simulink model "ev"  (R2021a)
settings: Solver=ode4  StartTime=0  StopTime=1082  FixedStep=sim_dt  RelTol=1e-3
model workspace (MAT data in the model file):
  T_eff_bp = [-270; -210; -150; -90; -30; 30; 90; 150; 210; 270]
  T_eff_bp_2 = [-270; -210; -150; -90; -30; 30; 90; 150; 210; 270]
  losses_table = [108927.107777 7820.2782368 7820.17609997 7820.2782368 7820.2782368 7820.2782368 7820.2782368 7820.26172359 7820.2782368 9345.38006027 108927.107777 7820.2782368 ... (100 elements, 10x10)]
  losses_table_2 = [108927.107777 7820.2782368 7820.17609997 7820.2782368 7820.2782368 7820.2782368 7820.2782368 7820.26172359 7820.2782368 9345.38006027 108927.107777 7820.2782368 ... (100 elements, 10x10)]
  w_eff_bp = [0; 888.888888889; 1777.77777778; 2666.66666667; 3555.55555556; 4444.44444444; 5333.33333333; 6222.22222222; 7111.11111111; 8000]
  w_eff_bp_2 = [0; 888.888888889; 1777.77777778; 2666.66666667; 3555.55555556; 4444.44444444; 5333.33333333; 6222.22222222; 7111.11111111; 8000]
undefined symbols (not defined in the file): Af, alpha, Bt, C, C_fa, C_free, C_sa_bat, C_sa_uc, Cd, Cmax, Continuous, Crr, DoD, effi, etaFD, etaG, FD, G, gear, Iucmax, m, M1m, M2m, Max, npar, npar_free, npara, nparf, nparfa, nparsa_bat, nparsa_UC, nser, nser_free, nserfa, nsersa_bat, nsersa_UC, Qbat, regenmax, Ri_BP, RL, ro, Rsc, Rsc_A, Rsc_F, Rsc_sa_bat, Rsc_sa_uc, rw, sim_dt, SOC_BP, SoCbatmax, SoCbatmin, SoCucmax, SoCucmin, speed, torque, VinBat, Voc_BP, Vuc, Vuc_fa, Vuc_free ... (+2)
libraries: autolibshared x41, simulink x26, autolibdcdc x13, autolibdatasheetbattery x7, autolibmappedmotor x6, fl_lib x3, nesl_utility x3, spsSupercapacitorLib x3, pid_lib x1
(part 18 of 18)

== matlab function ev/Drive cycle power demand/Controller. Actual motor torque/MATLAB Function ==
  data: trq_wh input; g1 output; w_wh input; P_veh input; Tau_def output; G parameter; effi parameter; speed parameter; torque parameter; etaG parameter; WG_def output; g0 input; gs output; Max parameter; Tmax output; Tmin output; Continuous parameter; g_prev input; n_mtr output; com output; test input; WG output; Vtest input; mode input; FD parameter; etaFD parameter; regenmax parameter
function [g1,Tau_def,WG_def,gs,Tmax,Tmin,n_mtr,com,WG] = fcn(trq_wh,w_wh,P_veh,G,effi, speed, torque,etaG,g0, Max,Continuous,g_prev,test,Vtest,mode,FD,etaFD,regenmax)



Wgb_out=w_wh.*FD;


WG=Wgb_out.*G; %Vel angular despues del Gear, ws intech velocidad angular de la flecha del motor el�ctrico ecuaci�n 8

WG(WG>max(Continuous(:,1))*pi/30)=max(Continuous(:,1))*pi/30;







    if P_veh>0
            Tgb_out=(1/etaFD)*trq_wh./(FD);
            Tau=(1/etaG)*Tgb_out./(G); %torque mecánico del motor electrico
                
           n_mtr=interp2(speed*(2*pi/60),-torque,effi,WG,Tau);
           if mode == 0 % for now the selection is only available with accel profile
            
            [com,gs]=min(WG); %for high performance mode 
           else
            [com,gs]=max(n_mtr); %for eco mode
           end
    else
            Tgb_out=(etaFD)*trq_wh./(FD);
            Tau=(etaG)*Tgb_out./(G);%torque mecnánico del generador electrico
                Tau(Tau<regenmax)=regenmax;
            n_mtr=interp2(speed*(2*pi/60),-torque,effi,WG,Tau);
            [com,gs]=max(n_mtr);
            
            
    %          gs=g_prev;
    %          com=n_mtr(:,gs);
    end

test1=all(test);

    if test1==1 % si los 30 anteriores son iguales

            if com==0
        
                gs=g_prev;
                WG_def=WG(gs);
                Tau_def=Tau(gs);
            else
                if Vtest==1 && g_prev>gs
                    
                    
                    gs=g_prev;
                    WG_def=WG(gs);
                    Tau_def=Tau(gs);
                else
                    gs=gs;
                    WG_def=WG(gs);
                    Tau_def=Tau(gs);
                end
            end
    Tmax=interp1(Continuous(:,1),Continuous(:,2),abs(WG_def)*(30/pi));
    Tmin=interp1(Continuous(:,1),-Continuous(:,2),abs(WG_def)*(30/pi));

    % Tcmax=interp1(Continuous(:,1),Continuous(:,2),WG_def*(30/pi));
    % Tcmin=interp1(Continuous(:,1),-Continuous(:,2),abs(WG_def)*(30/pi));

%         if     gs==1; 
%             g1=G(1);
%         elseif gs==2; 
%             g1=G(2);
% %         elseif gs==3; 
% %             g1=G(3);
% %         elseif gs==4; 
% %             g1=G(4);
% %         elseif gs==5; 
% %             g1=G(5);
% %         elseif gs==6; 
% %             g1=G(6);
% %         elseif gs==7; 
% %             g1=G(7);
% %         elseif gs==8; 
% %             g1=G(8); 
% %         else
%             g1=G(1);
%         end
        
%             g1=G(gs);
    else  %si el cambio de velocidad no ha sido constante los ultimos 30 dt
        gs=g_prev;
        WG_def=WG(gs);
        Tau_def=Tau(gs);  

    Tmax=interp1(Continuous(:,1),Continuous(:,2),abs(WG_def)*(30/pi));
    Tmin=interp1(Continuous(:,1),-Continuous(:,2),abs(WG_def)*(30/pi));

    % Tcmax=interp1(Continuous(:,1),Continuous(:,2),WG_def*(30/pi));
    % Tcmin=interp1(Continuous(:,1),-Continuous(:,2),abs(WG_def)*(30/pi));

%         if     gs==1; 
%             g1=G(1);
%         elseif gs==2; 
%             g1=G(2);
% %         elseif gs==3; 
% %             g1=G(3);
% %         elseif gs==4; 
% %             g1=G(4);
% %         elseif gs==5; 
% %             g1=G(5);
% %         elseif gs==6; 
% %             g1=G(6);
% %         elseif gs==7; 
% %             g1=G(7);
% %         elseif gs==8; 
% %             g1=G(8); 
%         else
%             g1=G(1);
%         end

            g1=G(gs);

    end
    
    
    
    
    

end

== matlab function ev/Tesis/HESS/Full active4/MATLAB Function3 ==
  data: Id output; Vo input; Vd input; eff input; Po input; Pd output; Io output
function [Id,Pd,Io]  = fcn(Vo,Vd,eff, Po)

if Po>0
    Pd=Po;
    Id=Pd/Vd;
    Io=Po/Vo;
elseif Po<0
    Pd=Po;
    Id=Pd/Vd;
    Io=Po/Vo;
else
    Pd=Po;
    Id=Pd/Vd;
    Io=Po/Vo;
end
   

end

== matlab function ev/Tesis/HESS/Full_active/MATLAB Function2 ==
  data: OCV input; I_batt output; Ri input; P input
function I_batt   = fcn(OCV,Ri,P)

%I_batt=(-OCV-sqrt((OCV^2)-(4*(-Ri)*(-P))))/(2*(-Ri));

I_batt=(-(OCV-(OCV^2-4*P*Ri)^(1/2))/(2*Ri));

% I_batt=roots([Ri -OCV P]);
% imIb=imag(I_batt);
% I_batt=min(imIb)
end

== matlab function ev/Tesis/HESS/Full active4/MATLAB Function5 ==
  data: Id output; Vo input; Vd input; eff input; Po input; Pd output; Io output
function [Id,Pd,Io]  = fcn(Vo,Vd,eff, Po)


    Pd=Po;
    Id=Pd/Vd;
    Io=Po/Vo;

   

end

== matlab function ev/Tesis/HESS/semi_active_UC/MATLAB Function ==
  data: Ireq output; Iout output; Preq input; V_bat input; V_uc input; Ibat output; Iuc output; SoCbat input; SoCuc input; err output; stop output; test input; flagpow output; mode output; convDCDC input; conDCDC input; Qbat parameter; nparsa_UC parameter; Iucmax parameter; npara parameter; SoCbatmin parameter; SoCucmin parameter; SoCbatmax parameter; SoCucmax parameter; Cmax parameter; Pdispm output; Pdispn output
function [Ireq,Iout,Ibat,Iuc,err,stop,flagpow,mode,Pdispm,Pdispn] = fcn(Preq,V_bat,V_uc,SoCbat,SoCuc,test,convDCDC,conDCDC,Qbat, nparsa_UC, Iucmax, npara, SoCbatmin, SoCucmin, SoCbatmax, SoCucmax,Cmax)

% if V_bat==V_uc
    V_tot=V_bat;
% else
%     V_tot=V_uc;
% end


Ireq=(Preq/V_tot);

Ibatdis=Qbat*nparsa_UC*Cmax;
Ibatcha=-Qbat*nparsa_UC*Cmax;

Pbatcha=Ibatcha*V_bat;%*convDCDC;
Pbatdis=Ibatdis*V_bat;%*convDCDC;

Iucdis=Iucmax*npara;
Iuccha=-Iucmax*npara;

Puccha=Iuccha*V_uc;%*conDCDC;
Pucdis=Iucdis*V_uc;%*conDCDC;

Pdispm=Pbatdis+Pucdis;
Pdispn=Pbatcha+Puccha;


   if Preq==0
       mode=0;
   elseif Preq>0
       if Preq<=(Pucdis+Pbatdis)
          if SoCbat<=SoCbatmin
              if SoCuc<=SoCucmin
                  mode=1;
              else
                  if Iucdis*convDCDC>=Ireq
                      mode=2;
                  else
                      mode=3;
                  end
              end
          else
              if SoCuc<=SoCucmin
                  if Ibatdis*convDCDC>=Ireq
                      mode=4;
                  else
                      mode=5;
                  end
              else
                  if test>0
                      if Iucdis*conDCDC>=Ireq
                          mode=6;
                      else
                          mode=7;
                      end
                  elseif test<0
                      if Ibatdis*convDCDC>=Ireq
                          mode=8;
                      else
                          mode=9;
                      end
                  else
                      mode=25;
                  end
              end
          end
       else
           if SoCbat<=SoCbatmin
               if SoCuc<=SoCucmin
                   mode=10;
               else
                   mode=11;
               end
           else
               if SoCuc<=SoCucmin
                   mode=12;
               else
                   mode=13;
               end
           end
       end
   elseif Preq<0
       if Preq>=(Pdispn)
           if SoCuc<=SoCucmax
               if SoCbat<=SoCbatmax
                   if Iuccha*conDCDC>=Ireq
                       mode=14;
                   else
                       mode=15;
                   end
               else
                   if Iuccha*conDCDC>Ireq
                       mode=16;
                   else
                       mode=17;
                   end
               end
           else
               if SoCbat<=SoCbatmax
                   if Ibatcha*convDCDC>Ireq
                       mode=18;
                   else
                       mode=19;
                   end
               else
                   mode=20;
               end
           end
       else
           if SoCuc<=SoCucmax
               if SoCbat<=SoCbatmax
                   mode=21;
               else
                   mode=22;
               end
           else
               if SoCbat<=SoCbatmax
                   mode=23;
               else
                   mode=24;
               end
           end
       end
   else
       mode=26;
   end
   
   switch mode
       case 0
           Iuc=0;
           Ibat=0;
           stop=0;
           err=0;
           flagpow=0;           
       case 1
           Iuc=0;
           Ibat=0;
           stop=1;
           err=0;
           flagpow=0;
       case 2
           Iuc=Ireq;
           Ibat=0;
           stop=0;
           err=0;
           flagpow=0;
       case 3
           Iuc=Iucdis*conDCDC;
           Ibat=0;
           stop=0;
           err=0;
           flagpow=1;
       case 4
           Iuc=Ireq-Ibatdis*convDCDC;
           Ibat=Ibatdis*convDCDC;
           stop=0;
           err=0;
           flagpow=0;
       case 5
           Iuc=0;
           Ibat=Ibatdis*convDCDC;
           stop=0;
           err=0;
           flagpow=1;
       case 6
           Iuc=Ireq;
           Ibat=0;
           stop=0;
           err=0;
           flagpow=0;
       case 7
           Iuc=Iucdis*conDCDC;
           Ibat=Ireq-Iucdis*conDCDC;
           stop=0;
           err=0;
           flagpow=0;
       case 8
           Iuc=Ireq-Ibatdis*convDCDC;
           Ibat=Ibatdis*convDCDC;
           stop=0;
           err=0;
           flagpow=0;
       case 9
           Iuc=0;
           Ibat=Ibatdis*convDCDC;
           stop=0;
           err=0;
           flagpow=1;
       case 10
           Iuc=0;
           Ibat=0;
           stop=1;
           err=0;
           flagpow=1;
       case 11
           Iuc=Iucdis*conDCDC;
           Ibat=0;
           stop=0;
           err=0;
           flagpow=1;
       case 12
           Iuc=0;
           Ibat=Ibatdis*convDCDC;
           stop=0;
           err=0;
           flagpow=1;
       case 13
           Iuc=Iucdis*conDCDC;
           Ibat=Ibatdis*convDCDC;
           stop=0;
           err=0;
           flagpow=1;
       case 14
           Iuc=Iuccha*conDCDC;;
           Ibat=Ireq-Iuccha*conDCDC;
           stop=0;
           err=0;
           flagpow=0;
       case 15 %mod
           Iuc=Ireq;
           Ibat=0;
           stop=0;
           err=0;
           flagpow=0;
       case 16
           Iuc=Iuccha*conDCDC;
           Ibat=0;
           stop=0;
           err=0;
           flagpow=1;
       case 17
           Iuc=Ireq;
           Ibat=0;
           stop=0;
           err=0;
           flagpow=0;
       case 18
           Iuc=0;
           Ibat=Ibatcha*convDCDC;
           stop=0;
           err=0;
           flagpow=0;
       case 19 %mod
           Iuc=0;
           Ibat=Ireq;
           stop=0;
           err=0;
           flagpow=0;
       case 20
           Iuc=0;
           Ibat=0;
           stop=0;
           err=0;
           flagpow=1;
       case 21
           Iuc=Iuccha*conDCDC;
           Ibat=Ibatcha*convDCDC;
           stop=0;
           err=0;
           flagpow=1;
       case 22
           Iuc=Iuccha*conDCDC;
           Ibat=0;
           stop=0;
           err=0;
           flagpow=1;
       case 23
           Iuc=0;
           Ibat=Ibatcha*convDCDC;
           stop=0;
           err=0;
           flagpow=1;
       case 24
           Iuc=0;
           Ibat=0;
           stop=0;
           err=0;
           flagpow=1;
       case 25 %case when count is 0
           Iuc=0;
           Ibat=0;
           stop=0;
           err=1;
           flagpow=0;
       case 26 %¿? it should not exist
           Iuc=0;
           Ibat=0;
           stop=0;
           err=2;
           flagpow=0;
       otherwise
           Iuc=0;
           Ibat=0;
           stop=0;
           err=3;
           flagpow=0;
           mode=27;
   end
   Iuc=Iuc*1;
   Ibat=Ibat*1;
Iout=Iuc+Ibat;

end

== matlab function ev/Tesis/HESS/semi_active_bat/MATLAB Function1 ==
  data: SoCuc input; acurr output; bcurr output; mo1 output; mo2 output; aprev input; bprev input; count output; cprev input; a output; b output; test output; counta output; countb output; cpreva input; cprevb input; countc output
function [acurr,bcurr,mo1,mo2,count,a,b,test,counta,countb,countc] = fcn(SoCuc,aprev,bprev,cprev,cpreva,cprevb)

if SoCuc>=0.2
    acurr=0;
    mo1=1;
else
    acurr=1;
    mo1=2;
end
if SoCuc>=0.9
    bcurr=1;
    mo2=1;
else
    bcurr=0;
    mo2=2;
end

a=acurr-aprev;
b=bcurr-bprev;




if a==1 || b==1
%     count=cprev+a+b;
    counta=cpreva+a;
    countb=cprevb+b;
else
%     count=cprev;
    counta=cpreva;
    countb=cprevb;
end
countc=countb-counta;

if countc>0
    count=2;
else 
    count=1;
end

test=(-1)^(count);

end

== matlab function ev/Tesis/HESS/semi_active_UC/MATLAB Function2 ==
  data: OCV input; I_batt output; Ri input; P input
function I_batt   = fcn(OCV,Ri,P)

%I_batt=(-OCV-sqrt((OCV^2)-(4*(-Ri)*(-P))))/(2*(-Ri));

I_batt=(-(OCV-(OCV^2-4*P*Ri)^(1/2))/(2*Ri));

% I_batt=roots([Ri -OCV P]);
% imIb=imag(I_batt);
% I_batt=min(imIb)
end

== matlab function ev/Tesis/HESS/semi_active_UC/MATLAB Function3 ==
  data: Id output; Vo input; Vd input; eff input; Po input; Pd output; Io output
function [Id,Pd,Io]  = fcn(Vo,Vd,eff, Po)

if Po>0
    Pd=Po;
    Id=Pd/Vd;
    Io=Po/Vo;
elseif Po<0
    Pd=Po;
    Id=Pd/Vd;
    Io=Po/Vo;
else
    Pd=Po;
    Id=Pd/Vd;
    Io=Po/Vo;
end
   

end

== matlab function ev/Tesis/HESS/semi_active_bat/MATLAB Function ==
  data: Ireq output; Iout output; Preq input; V_bat input; V_uc input; Ibat output; Iuc output; SoCbat input; SoCuc input; err output; stop output; test input; flagpow output; mode output; convDCDC input; conDCDC input; Qbat parameter; nparsa_bat parameter; Iucmax parameter; nparf parameter; SoCucmin parameter; SoCbatmin parameter; SoCbatmax parameter; SoCucmax parameter; Cmax parameter
function [Ireq,Iout,Ibat,Iuc,err,stop,flagpow,mode] = fcn(Preq,V_bat,V_uc,SoCbat,SoCuc,test,convDCDC,conDCDC,Qbat, nparsa_bat, Iucmax, nparf, SoCucmin, SoCbatmin, SoCbatmax, SoCucmax,Cmax)

% if V_bat==V_uc
%     V_tot=V_bat;
% else
    V_tot=V_uc;
% end


Ireq=(Preq/V_tot);

Ibatdis=Qbat*nparsa_bat*Cmax;
Ibatcha=-Qbat*nparsa_bat*Cmax;

Pbatcha=Ibatcha*V_bat;%*convDCDC;
Pbatdis=Ibatdis*V_bat;%*convDCDC;

Iucdis=Iucmax*nparf;
Iuccha=-Iucmax*nparf;

Puccha=Iuccha*V_uc;%*conDCDC;
Pucdis=Iucdis*V_uc;%*conDCDC;




   if Preq==0
       mode=0;
   elseif Preq>0
       if Preq<=(Pucdis+Pbatdis)
          if SoCbat<=SoCbatmin
              if SoCuc<=SoCucmin
                  mode=1;
              else
                  if Iucdis*convDCDC>=Ireq
                      mode=2;
                  else
                      mode=3;
                  end
              end
          else
              if SoCuc<=SoCucmin
                  if Ibatdis*convDCDC>=Ireq
                      mode=4;
                  else
                      mode=5;
                  end
              else
                  if test>0
                      if Iucdis*conDCDC>=Ireq
                          mode=6;
                      else
                          mode=7;
                      end
                  elseif test<0
                      if Ibatdis*convDCDC>=Ireq
                          mode=8;
                      else
                          mode=9;
                      end
                  else
                      mode=25;
                  end
              end
          end
       else
           if SoCbat<=SoCbatmin
               if SoCuc<=SoCucmin
                   mode=10;
               else
                   mode=11;
               end
           else
               if SoCuc<=SoCucmin
                   mode=12;
               else
                   mode=13;
               end
           end
       end
   elseif Preq<0
       if Preq>=(Puccha+Pbatcha)
           if SoCuc<=SoCucmax
               if SoCbat<=SoCbatmax
                   if Iuccha*conDCDC>Ireq
                       mode=14;
                   else
                       mode=15;
                   end
               else
                   if Iuccha*conDCDC>Ireq
                       mode=16;
                   else
                       mode=17;
                   end
               end
           else
               if SoCbat<=SoCbatmax
                   if Ibatcha*convDCDC>Ireq
                       mode=18;
                   else
                       mode=19;
                   end
               else
                   mode=20;
               end
           end
       else
           if SoCuc<=SoCucmax
               if SoCbat<=SoCbatmax
                   mode=21;
               else
                   mode=22;
               end
           else
               if SoCbat<=SoCbatmax
                   mode=23;
               else
                   mode=24;
               end
           end
       end
   else
       mode=26;
   end
   
   switch mode
       case 0
           Iuc=0;
           Ibat=0;
           stop=0;
           err=0;
           flagpow=0;           
       case 1
           Iuc=0;
           Ibat=0;
           stop=1;
           err=0;
           flagpow=0;
       case 2
           Iuc=Ireq;
           Ibat=0;
           stop=0;
           err=0;
           flagpow=0;
       case 3
           Iuc=Iucdis*conDCDC;
           Ibat=0;
           stop=0;
           err=0;
           flagpow=1;
       case 4
           Iuc=Ireq-Ibatdis*convDCDC;
           Ibat=Ibatdis*convDCDC;
           stop=0;
           err=0;
           flagpow=0;
       case 5
           Iuc=0;
           Ibat=Ibatdis*convDCDC;
           stop=0;
           err=0;
           flagpow=1;
       case 6
           Iuc=Ireq;
           Ibat=0;
           stop=0;
           err=0;
           flagpow=0;
       case 7
           Iuc=Iucdis*conDCDC;
           Ibat=Ireq-Iucdis*conDCDC;
           stop=0;
           err=0;
           flagpow=0;
       case 8
           Iuc=Ireq-Ibatdis*convDCDC;
           Ibat=Ibatdis*convDCDC;
           stop=0;
           err=0;
           flagpow=0;
       case 9
           Iuc=0;
           Ibat=Ibatdis*convDCDC;
           stop=0;
           err=0;
           flagpow=1;
       case 10
           Iuc=0;
           Ibat=0;
           stop=1;
           err=0;
           flagpow=1;
       case 11
           Iuc=Iucdis*conDCDC;
           Ibat=0;
           stop=0;
           err=0;
           flagpow=1;
       case 12
           Iuc=0;
           Ibat=Ibatdis*convDCDC;
           stop=0;
           err=0;
           flagpow=1;
       case 13
           Iuc=Iucdis*conDCDC;
           Ibat=Ibatdis*convDCDC;
           stop=0;
           err=0;
           flagpow=1;
       case 14
           Iuc=Iuccha*conDCDC;;
           Ibat=Ireq-Iuccha*conDCDC;
           stop=0;
           err=0;
           flagpow=0;
       case 15 %mod
           Iuc=Ireq;
           Ibat=0;
           stop=0;
           err=0;
           flagpow=0;
       case 16
           Iuc=Iuccha*conDCDC;
           Ibat=0;
           stop=0;
           err=0;
           flagpow=1;
       case 17
           Iuc=Ireq;
           Ibat=0;
           stop=0;
           err=0;
           flagpow=0;
       case 18
           Iuc=0;
           Ibat=Ibatcha*convDCDC;
           stop=0;
           err=0;
           flagpow=0;
       case 19 %mod
           Iuc=0;
           Ibat=Ireq;
           stop=0;
           err=0;
           flagpow=0;
       case 20
           Iuc=0;
           Ibat=0;
           stop=0;
           err=0;
           flagpow=1;
       case 21
           Iuc=Iuccha*conDCDC;
           Ibat=Ibatcha*convDCDC;
           stop=0;
           err=0;
           flagpow=1;
       case 22
           Iuc=Iuccha*conDCDC;
           Ibat=0;
           stop=0;
           err=0;
           flagpow=1;
       case 23
           Iuc=0;
           Ibat=Ibatcha*convDCDC;
           stop=0;
           err=0;
           flagpow=1;
       case 24
           Iuc=0;
           Ibat=0;
           stop=0;
           err=0;
           flagpow=1;
       case 25 %case when count is 0
           Iuc=0;
           Ibat=0;
           stop=0;
           err=1;
           flagpow=0;
       case 26 %¿? it should not exist
           Iuc=0;
           Ibat=0;
           stop=0;
           err=2;
           flagpow=0;
       otherwise
           Iuc=0;
           Ibat=0;
           stop=0;
           err=3;
           flagpow=0;
           mode=27;
   end
   Iuc=Iuc*1;
   Ibat=Ibat*1;
Iout=Iuc+Ibat;

end

== matlab function ev/Tesis/HESS/Free/MATLAB Function ==
  data: Ireq output; Iout output; Preq input; V_bat input; V_uc input; Ibat output; I_uc output; SoCbat input; SoCuc input; err output; stop output; test input; flagpow output; mode output; convDCDC input; conDCDC input; Qbat parameter; npar_free parameter; Iucmax parameter; nparf parameter; SoCbatmin parameter; SoCucmin parameter; SoCbatmax parameter; SoCucmax parameter
function [Ireq,Iout,Ibat,I_uc,err,stop,flagpow,mode] = fcn(Preq,V_bat,V_uc,SoCbat,SoCuc,test,convDCDC,conDCDC,Qbat, npar_free, Iucmax, nparf, SoCbatmin, SoCucmin, SoCbatmax, SoCucmax)


    V_tot=V_bat;



Ireq=(Preq/V_tot);

Ibatdis=Qbat*npar_free;
Ibatcha=-Qbat*npar_free;

Pbatcha=Ibatcha*V_tot;%*convDCDC;
Pbatdis=Ibatdis*V_tot;%*convDCDC;

Iucdis=Iucmax*nparf;
Iuccha=-Iucmax*nparf;

Puccha=Iuccha*V_tot;%*conDCDC;
Pucdis=Iucdis*V_tot;%*conDCDC;



   
if V_bat==V_uc
        I_uc=Ireq/2;
        Ibat=Ireq/2;
        stop=0;
        err=0;
        flagpow=0;
        mode=0;
elseif V_bat>V_uc
        if Preq>=0
            if Preq<Pbatdis
            I_uc=Ireq-Ibatdis;
            Ibat=Ibatdis;
            stop=0;
            err=0;
            flagpow=0;
            mode=1;
            else
            I_uc=0;
            Ibat=Ibatdis;
            stop=0;
            err=0;
            flagpow=1;
            mode=2;
            end
        else  %si la potencia requerida es menor a cero
            if Preq<Puccha
            I_uc=Iuccha;
            Ibat=Ireq-Iuccha;
            stop=0;
            err=0;
            flagpow=0;
            mode=3;
            else
            I_uc=Ireq;
            Ibat=0;
            stop=0;
            err=0;
            flagpow=1;
            mode=4;
            end
        end
elseif V_bat<V_uc
        if Preq>0
            if Preq<=Pucdis  %la potencia total la puede dar el UC, tambien puede cargar la bateria
            I_uc=Ireq;
            Ibat=0;
            stop=0;
            err=0;
            flagpow=0;
            mode=5;
            else
            I_uc=Iucdis;
            Ibat=Ireq-Iucdis;
            stop=0;
            err=0;
            flagpow=1;
            mode=6;
            end
        elseif Preq<0
            if Preq<Puccha
            I_uc=Iuccha;
            Ibat=Ireq-Iuccha;
            stop=0;
            err=0;
            flagpow=0;
            mode=7;
            else
            I_uc=Ireq;
            Ibat=0;
            stop=0;
            err=0;
            flagpow=1;
            mode=8;
            end
        else
            I_uc=0;
            Ibat=0;
            stop=0;
            err=0;
            flagpow=0;
            mode=9;
        end
else
        I_uc=0;
        Ibat=0;
        stop=0;
        err=1;
        flagpow=0;
        mode=10;
    
end

    I_uc=I_uc*1;
    Ibat=Ibat*1;
    Iout=I_uc+Ibat;


end

== matlab function ev/Tesis/HESS/semi_active_bat/MATLAB Function2 ==
  data: OCV input; I_batt output; Ri input; P input
function I_batt   = fcn(OCV,Ri,P)

%I_batt=(-OCV-sqrt((OCV^2)-(4*(-Ri)*(-P))))/(2*(-Ri));

I_batt=(-(OCV-(OCV^2-4*P*Ri)^(1/2))/(2*Ri));

% I_batt=roots([Ri -OCV P]);
% imIb=imag(I_batt);
% I_batt=min(imIb)
end

== matlab function ev/Tesis/HESS/semi_active_UC/MATLAB Function4 ==
  data: SoCuc input; acurr output; bcurr output; mo1 output; mo2 output; aprev input; bprev input; count output; cprev input; a output; b output; test output; counta output; countb output; cpreva input; cprevb input; countc output
function [acurr,bcurr,mo1,mo2,count,a,b,test,counta,countb,countc] = fcn(SoCuc,aprev,bprev,cprev,cpreva,cprevb)

if SoCuc>=0.2
    acurr=0;
    mo1=1;
else
    acurr=1;
    mo1=2;
end
if SoCuc>=0.9
    bcurr=1;
    mo2=1;
else
    bcurr=0;
    mo2=2;
end

a=acurr-aprev;
b=bcurr-bprev;




if a==1 || b==1
%     count=cprev+a+b;
    counta=cpreva+a;
    countb=cprevb+b;
else
%     count=cprev;
    counta=cpreva;
    countb=cprevb;
end
countc=countb-counta;

if countc>0
    count=2;
else 
    count=1;
end

test=(-1)^(count);

end

== matlab function ev/Tesis/HESS/semi_active_bat/MATLAB Function5 ==
  data: Id output; Vo input; Vd input; eff input; Po input; Pd output; Io output
function [Id,Pd,Io]  = fcn(Vo,Vd,eff, Po)

if Po>0
    Pd=Po;
    Id=Pd/Vd;
    Io=Po/Vo;
elseif Po<0
    Pd=Po;
    Id=Pd/Vd;
    Io=Po/Vo;
else
    Pd=Po;
    Id=Pd/Vd;
    Io=Po/Vo;
end
   

end

== matlab function ev/Tesis/HESS/Free/MATLAB Function1 ==
  data: SoCuc input; acurr output; bcurr output; mo1 output; mo2 output; aprev input; bprev input; count output; cprev input; a output; b output; test output; counta output; countb output; cpreva input; cprevb input; countc output
function [acurr,bcurr,mo1,mo2,count,a,b,test,counta,countb,countc] = fcn(SoCuc,aprev,bprev,cprev,cpreva,cprevb)

if SoCuc>=0.2
    acurr=0;
    mo1=1;
else
    acurr=1;
    mo1=2;
end
if SoCuc>=0.9
    bcurr=1;
    mo2=1;
else
    bcurr=0;
    mo2=2;
end

a=acurr-aprev;
b=bcurr-bprev;




if a==1 || b==1
%     count=cprev+a+b;
    counta=cpreva+a;
    countb=cprevb+b;
else
%     count=cprev;
    counta=cpreva;
    countb=cprevb;
end
countc=countb-counta;

if countc>0
    count=2;
else 
    count=1;
end

test=(-1)^(count);

end

== matlab function ev/Tesis/HESS/Free/MATLAB Function2 ==
  data: OCV input; I_batt output; Ri input; P input
function I_batt   = fcn(OCV,Ri,P)

%I_batt=(-OCV-sqrt((OCV^2)-(4*(-Ri)*(-P))))/(2*(-Ri));

I_batt=(-(OCV-(OCV^2-4*P*Ri)^(1/2))/(2*Ri));

% I_batt=roots([Ri -OCV P]);
% imIb=imag(I_batt);
% I_batt=min(imIb)
end

== matlab function ev/Tesis/HESS/semi_active_bat/vehicle dynamics/MATLAB Function ==
  data: F_FA input; F_veh input; igu input; u output; velo input; z1 input; a output
function [u,a]  = fcn(F_FA,F_veh,igu,velo,z1)




if (F_FA-F_veh)<3 && (F_FA-F_veh)> (-3) 
    
    u=velo;
    a=1;
else
    a=0;
    u=z1;
end






end

== matlab function ev/Tesis/HESS/semi_active_UC/vehicle dynamics/MATLAB Function ==
  data: F_FA input; F_veh input; igu input; u output; velo input; z1 input; a output
function [u,a]  = fcn(F_FA,F_veh,igu,velo,z1)




if (F_FA-F_veh)<3 && (F_FA-F_veh)> (-3) 
    
    u=velo;
    a=1;
else
    a=0;
    u=z1;
end






end

== matlab function ev/Tesis/HESS/Full_active/vehicle dynamics/MATLAB Function ==
  data: F_FA input; F_veh input; igu input; u output; velo input; z1 input; a output
function [u,a]  = fcn(F_FA,F_veh,igu,velo,z1)




if (F_FA-F_veh)<3 && (F_FA-F_veh)> (-3) 
    
    u=velo;
    a=1;
else
    a=0;
    u=z1;
end






end

== matlab function ev/Tesis/HESS/Free/vehicle dynamics/MATLAB Function ==
  data: F_FA input; F_veh input; igu input; u output; velo input; z1 input; a output
function [u,a]  = fcn(F_FA,F_veh,igu,velo,z1)




if (F_FA-F_veh)<3 && (F_FA-F_veh)> (-3) 
    
    u=velo;
    a=1;
else
    a=0;
    u=z1;
end






end

== matlab function ev/Tesis/Battery model/MATLAB Function1 ==
  data: Ri input; Vb output; Ib input; Pmot input
function Vb = fcn(Ri,Ib,Pmot)

Vb=(((Ri*(Ib^2))+Pmot)/(Ib));


end

== matlab function ev/battery model limited/MATLAB Function ==
  data: OCV input; I_batt output; Ri input; P input
function I_batt   = fcn(OCV,Ri,P)

%I_batt=(-OCV-sqrt((OCV^2)-(4*(-Ri)*(-P))))/(2*(-Ri));

I_batt=(-(OCV-(OCV^2-4*P*Ri)^(1/2))/(2*Ri));

% I_batt=roots([Ri -OCV P]);
% imIb=imag(I_batt);
% I_batt=min(imIb)
end

== matlab function ev/battery model limited/MATLAB Function2 ==
  data: Ri input; Vb output; Ib input; Pmot input
function Vb = fcn(Ri,Ib,Pmot)

Vb=-(((Ri*(Ib^2))+Pmot)/(Ib));

Vb=Vb-Ri*Ib;

end

== matlab function ev/Tesis/HESS/Battery model/MATLAB Function1 ==
  data: Ri input; Vb output; Ib input; Pmot input
function Vb = fcn(Ri,Ib,Pmot)

Vb=(((Ri*(Ib^2))+Pmot)/(Ib));


end

== matlab function ev/Tesis/battery model limitedmod/MATLAB Function ==
  data: OCV input; I_batt output; Ri input; P input
function I_batt   = fcn(OCV,Ri,P)

%I_batt=(-OCV-sqrt((OCV^2)-(4*(-Ri)*(-P))))/(2*(-Ri));

I_batt=(-(OCV-(OCV^2-4*P*Ri)^(1/2))/(2*Ri));

% I_batt=roots([Ri -OCV P]);
% imIb=imag(I_batt);
% I_batt=min(imIb)
end

== matlab function ev/vehicle dynamics1/MATLAB Function ==
  data: F_FA input; F_veh input; igu input; u output; velo input; z1 input; a output
function [u,a]  = fcn(F_FA,F_veh,igu,velo,z1)




if (F_FA-F_veh)<3 && (F_FA-F_veh)> (-3) 
    
    u=velo;
    a=1;
else
    a=0;
    u=z1;
end






end

== matlab function ev/Tesis/Battery model/vehicle dynamics/MATLAB Function ==
  data: F_FA input; F_veh input; igu input; u output; velo input; z1 input; a output
function [u,a]  = fcn(F_FA,F_veh,igu,velo,z1)




if (F_FA-F_veh)<3 && (F_FA-F_veh)> (-3) 
    
    u=velo;
    a=1;
else
    a=0;
    u=z1;
end






end

== matlab function ev/Tesis/battery model limitedmod/MATLAB Function2 ==
  data: Ri input; Vb output; Ib input; Pmot input
function Vb = fcn(Ri,Ib,Pmot)

Vb=-(((Ri*(Ib^2))+Pmot)/(Ib));

Vb=Vb-Ri*Ib;

end

== matlab function ev/Tesis/HESS/battery model limited/MATLAB Function2 ==
  data: Ri input; Vb output; Ib input; Pmot input
function Vb = fcn(Ri,Ib,Pmot)

Vb=-(((Ri*(Ib^2))+Pmot)/(Ib));


end

== matlab function ev/Tesis/HESS/semi active Bat//Bat/MATLAB Function ==
  data: Ireq output; Iout output; Preq input; V_bat input; V_uc input; Ibat output; Iuc output; SoCbat input; SoCuc input; err output; stop output; test input; flagpow output; mode output; convDCDC input
function [Ireq,Iout,Ibat,Iuc,err,stop,flagpow,mode] = fcn(Preq,V_bat,V_uc,SoCbat,SoCuc,test,convDCDC)
conDCDC=1;
if V_bat==V_uc
    V_tot=V_bat;
else
    V_tot=V_uc;
end


Ireq=(Preq/V_tot);
Ibatdis=150;
Ibatcha=-150;
Pbatcha=Ibatcha*V_tot*convDCDC;
Pbatdis=Ibatdis*V_tot*convDCDC;
Iucdis=300;
Iuccha=-300;
Puccha=Iuccha*V_tot*conDCDC;
Pucdis=Iucdis*V_tot*conDCDC;


SoCbatmin=0.2;
SoCucmin=0.2;
SoCbatmax=0.85;
SoCucmax=0.95;




   if Preq==0
       mode=0;
   elseif Preq>0
       if Preq<=(Pucdis+Pbatdis)
          if SoCbat<=SoCbatmin
              if SoCuc<=SoCucmin
                  mode=1;
              else
                  if Iucdis>=Ireq
                      mode=2;
                  else
                      mode=3;
                  end
              end
          else
              if SoCuc<=SoCucmin
                  if Ibatdis*convDCDC>=Ireq
                      mode=4;
                  else
                      mode=5;
                  end
              else
                  if test>0
                      if Iucdis*conDCDC>=Ireq
                          mode=6;
                      else
                          mode=7;
                      end
                  elseif test<0
                      if Ibatdis*convDCDC>=Ireq
                          mode=8;
                      else
                          mode=9;
                      end
                  else
                      mode=25;
                  end
              end
          end
       else
           if SoCbat<=SoCbatmin
               if SoCuc<=SoCucmin
                   mode=10;
               else
                   mode=11;
               end
           else
               if SoCuc<=SoCucmin
                   mode=12;
               else
                   mode=13;
               end
           end
       end
   elseif Preq<0
       if Preq>=(Puccha+Pbatcha)
           if SoCuc<=SoCucmax
               if SoCbat<=SoCbatmax
                   if Iuccha*conDCDC>Ireq
                       mode=14;
                   else
                       mode=15;
                   end
               else
                   if Iuccha*conDCDC>Ireq
                       mode=16;
                   else
                       mode=17;
                   end
               end
           else
               if SoCbat<=SoCbatmax
                   if Ibatcha*convDCDC>Ireq
                       mode=18;
                   else
                       mode=19;
                   end
               else
                   mode=20;
               end
           end
       else
           if SoCuc<=SoCucmax
               if SoCbat<=SoCbatmax
                   mode=21;
               else
                   mode=22;
               end
           else
               if SoCbat<=SoCbatmax
                   mode=23;
               else
                   mode=24;
               end
           end
       end
   else
       mode=26;
   end
   
   switch mode
       case 0
           Iuc=0;
           Ibat=0;
           stop=0;
           err=0;
           flagpow=0;           
       case 1
           Iuc=0;
           Ibat=0;
           stop=1;
           err=0;
           flagpow=0;
       case 2
           Iuc=Ireq;
           Ibat=0;
           stop=0;
           err=0;
           flagpow=0;
       case 3
           Iuc=Iucdis*conDCDC;
           Ibat=0;
           stop=0;
           err=0;
           flagpow=1;
       case 4
           Iuc=Ireq-Ibatdis*convDCDC;
           Ibat=Ibatdis*convDCDC;
           stop=0;
           err=0;
           flagpow=0;
       case 5
           Iuc=0;
           Ibat=Ibatdis*convDCDC;
           stop=0;
           err=0;
           flagpow=1;
       case 6
           Iuc=Ireq;
           Ibat=0;
           stop=0;
           err=0;
           flagpow=0;
       case 7
           Iuc=Iucdis*conDCDC;
           Ibat=Ireq-Iucdis*conDCDC;
           stop=0;
           err=0;
           flagpow=0;
       case 8
           Iuc=Ireq-Ibatdis*convDCDC;
           Ibat=Ibatdis*convDCDC;
           stop=0;
           err=0;
           flagpow=0;
       case 9
           Iuc=0;
           Ibat=Ibatdis*convDCDC;
           stop=0;
           err=0;
           flagpow=1;
       case 10
           Iuc=0;
           Ibat=0;
           stop=1;
           err=0;
           flagpow=1;
       case 11
           Iuc=Iucdis*conDCDC;
           Ibat=0;
           stop=0;
           err=0;
           flagpow=1;
       case 12
           Iuc=0;
           Ibat=Ibatdis*convDCDC;
           stop=0;
           err=0;
           flagpow=1;
       case 13
           Iuc=Iucdis*conDCDC;
           Ibat=Ibatdis*convDCDC;
           stop=0;
           err=0;
           flagpow=1;
       case 14
           Iuc=Iuccha*conDCDC;
           Ibat=Ireq-Iuccha*conDCDC;
           stop=0;
           err=0;
           flagpow=0;
       case 15 %mod
           Iuc=0;
           Ibat=Ireq;
           stop=0;
           err=0;
           flagpow=0;
       case 16
           Iuc=Iuccha*conDCDC;
           Ibat=0;
           stop=0;
           err=0;
           flagpow=1;
       case 17
           Iuc=Ireq;
           Ibat=0;
           stop=0;
           err=0;
           flagpow=0;
       case 18
           Iuc=0;
           Ibat=Ibatcha*convDCDC;
           stop=0;
           err=0;
           flagpow=0;
       case 19 %mod
           Iuc=0;
           Ibat=Ireq;
           stop=0;
           err=0;
           flagpow=0;
       case 20
           Iuc=0;
           Ibat=0;
           stop=0;
           err=0;
           flagpow=1;
       case 21
           Iuc=Iuccha*conDCDC;
           Ibat=Ibatcha*convDCDC;
           stop=0;
           err=0;
           flagpow=1;
       case 22
           Iuc=Iuccha*conDCDC;
           Ibat=0;
           stop=0;
           err=0;
           flagpow=1;
       case 23
           Iuc=0;
           Ibat=Ibatcha*convDCDC;
           stop=0;
           err=0;
           flagpow=1;
       case 24
           Iuc=0;
           Ibat=0;
           stop=0;
           err=0;
           flagpow=1;
       case 25 %case when count is 0
           Iuc=0;
           Ibat=0;
           stop=0;
           err=1;
           flagpow=0;
       case 26 %¿? it should not exist
           Iuc=0;
           Ibat=0;
           stop=0;
           err=2;
           flagpow=0;
       otherwise
           Iuc=0;
           Ibat=0;
           stop=0;
           err=3;
           flagpow=0;
           mode=27
   end
   Iuc=Iuc*1;
   Ibat=Ibat*1;
Iout=Iuc+Ibat;

end
